simulink library "BicopLibrary"  (R2022b)
settings: Solver=VariableStepAuto  StartTime=0.0  StopTime=10.0  RelTol=1e-3
undefined symbols (not defined in the file or in its folder): Ts
libraries: arduinolib x7, $bdroot x3
settings Model: Creator=42190  LastModifiedBy=marti
settings DebuggingCC: UnconnectedInputMsg=warning  UnconnectedOutputMsg=warning  UnconnectedLineMsg=warning
settings ModelReferenceCC: EnableRefExpFcnMdlSchedulingChecks=on
settings RTWCC: DLArmComputeVersion=19.05

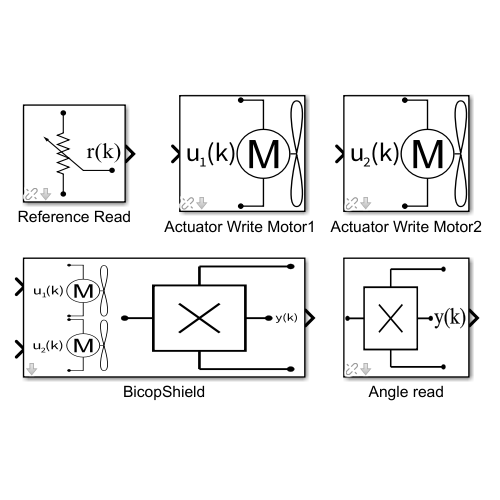
[thumbnail: Simulink's stored preview of the top-level diagram]
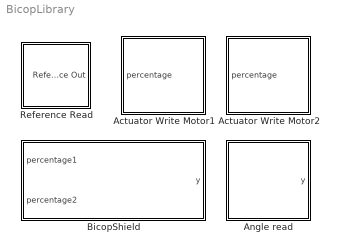
== system BicopLibrary ==
  "Actuator Write Motor1 " : Subsystem  AncestorBlock=BiCopLibrary/AeroShield/Actuator write
      settings: LibrarySourceBlock=BiCopLibrary/AeroShield/Actuator write
      mask DialogControl DescGroupVar Prompt: BicopShield actuator1
      mask DialogControl DescTextVar Prompt: Sets speed level to the first motor of the BicopShield. Expects input in form of percentual value from 0% to 100%.
      mask Display: image('$imagefile'); % Use "Edit Image" on toolstrip to change.
  Actuator Write Motor2 : Subsystem  AncestorBlock=BiCopLibrary/Actuator Write
      settings: LibrarySourceBlock=BiCopLibrary/Actuator Write
      mask DialogControl DescGroupVar Prompt: BicopShield actuator2
      mask DialogControl DescTextVar Prompt: Sets speed level to the second motor of the BicopShield. Expects input in form of percentual value from 0% to 100%.
      mask Display: image('$imagefile'); % Use "Edit Image" on toolstrip to change.
  Angle read : Subsystem  AncestorBlock=AeroLibrary/Angle read
      settings: LibrarySourceBlock=AeroLibrary/Angle read
      mask DialogControl DescGroupVar Prompt: BicopShield angle reading
      mask DialogControl DescTextVar Prompt: Sends commands to AS5600 sensor to read the pendulum angle. Output is in radians
      mask Display: image('$imagefile'); % Use "Edit Image" on toolstrip to change.
  BicopShield : Subsystem
      mask DialogControl DescGroupVar Prompt: BicopShield
      mask DialogControl DescTextVar Prompt: This block represents the BicopShield device. It accepts an input signal for powering the motors in the range of 0-100% and outputs a sensor angle reading in radians. Inside this system, you will find three subsystems. One of them reads the angle from sensor and the second one controls the BicopShield actuators respectively.
      mask Display: image('$imagefile'); % Use "Edit Image" on toolstrip to change.
  Reference Read : Subsystem  AncestorBlock=MotoLibrary/Reference Read
      settings: LibrarySourceBlock=MotoLibrary/Reference Read
      mask DialogControl DescGroupVar Prompt: BicopShield Potentiometer
      mask DialogControl DescTextVar Prompt: This blocks reads potentiometer wiper value on the BicopShield device. Return a percentage value.
      mask Display: image('$imagefile'); % Use "Edit Image" on toolstrip to change.

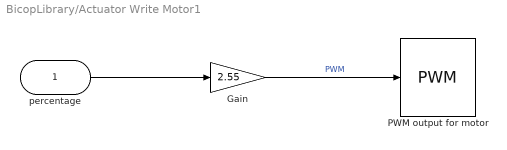
== system BicopLibrary/Actuator Write Motor1  ==
  percentage : Inport
  Gain : Gain  Gain=2.55
  "PWM output for motor " : arduinolib/PWM  pinNumber=5  frequencyType=Default  desiredFrequency=490.2  achievableFrequency=490.2
  wires:
  percentage/1 -> Gain/1
  Gain/1 -> "PWM output for motor "/1  "PWM"

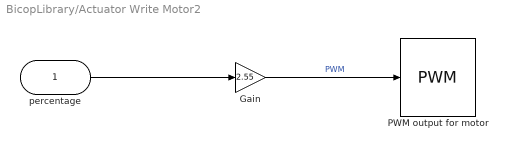
== system BicopLibrary/Actuator Write Motor2 ==
  percentage : Inport
  Gain : Gain  Gain=2.55
  "PWM output for motor " : arduinolib/PWM  pinNumber=6  frequencyType=Default  desiredFrequency=490.2  achievableFrequency=490.2
  wires:
  percentage/1 -> Gain/1
  Gain/1 -> "PWM output for motor "/1  "PWM"

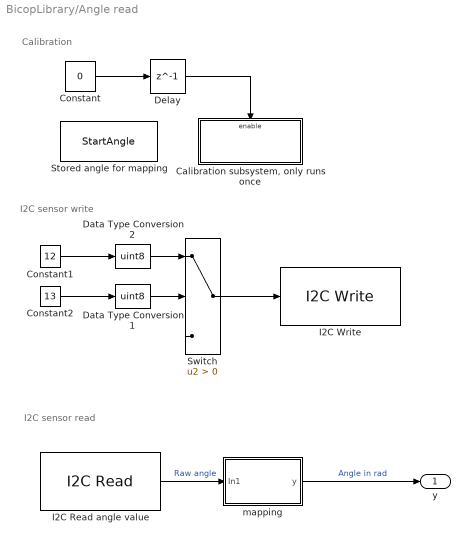
== system BicopLibrary/Angle read ==
  note: I2C sensor read
  note: I2C sensor write
  note: Calibration
  "Calibration subsystem, only runs once" : Subsystem  TreatAsAtomicUnit=on
  Constant : Constant  Value=0
  Constant1 : Constant  Value=12
  Constant2 : Constant  Value=13
  Data Type Conversion1 : DataTypeConversion  OutDataTypeStr=uint8  SaturateOnIntegerOverflow=off  RndMeth=Floor
  Data Type Conversion2 : DataTypeConversion  OutDataTypeStr=uint8  SaturateOnIntegerOverflow=off  RndMeth=Floor
  Delay : Delay  DelayLength=1  InitialCondition=1
  I2C Read angle value : arduinolib/I2C Read  I2CModule=0  Mode=Master  SlaveAddress=uint8(hex2dec('36'))  SlaveByteOrder=BigEndian  Direction=Receiver  RegisterAddressMode=off  RegisterAddress=uint8(hex2dec('36'))  SlaveDataType=uint16  DataLength=1  NoAck=off  RepeatedStart=off  OutputStatus=off  blockPlatform=ARDUINO  SampleTime=-1
  I2C Write : arduinolib/I2C Write  I2CModule=0  Mode=Master  SlaveAddress=uint8(hex2dec('36'))  SlaveByteOrder=BigEndian  Direction=Transmitter  RegisterAddressMode=off  RegisterAddress=uint8(hex2dec('0c'))  SlaveDataType=uint8  DataLength=1  NoAck=off  RepeatedStart=off  OutputStatus=off  blockPlatform=ARDUINO
  Stored angle for mapping : DataStoreMemory  DataStoreName=StartAngle  ReadBeforeWriteMsg=warning  WriteAfterWriteMsg=warning  WriteAfterReadMsg=warning  ShowAdditionalParam=off
  Switch : Switch  Criteria=u2 > Threshold  SaturateOnIntegerOverflow=off  InputSameDT=off
  mapping : Subsystem
  y : Outport
  wires:
  mapping/1(y) -> y/1  "Angle in rad"
  Constant/1 -> Delay/1
  Delay/1 -> "Calibration subsystem, only runs once"/Enable
  I2C Read angle value/1 -> mapping/1(In1)  "Raw angle"
  ? -> Switch/3
  Constant1/1 -> Data Type Conversion2/1
  Constant2/1 -> Data Type Conversion1/1
  Switch/1 -> I2C Write/1
  Data Type Conversion2/1 -> Switch/1
  Data Type Conversion1/1 -> Switch/2

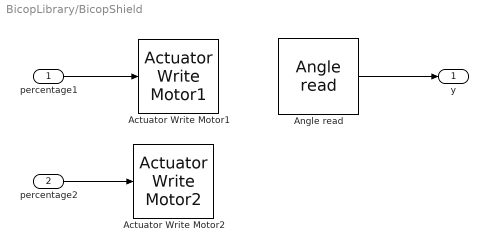
== system BicopLibrary/BicopShield ==
  percentage1 : Inport
  percentage2 : Inport  Port=2
  "Actuator Write Motor1 " : $bdroot/Actuator Write Motor1 
      settings: LibrarySourceBlock=BiCopLibrary/AeroShield/Actuator write
  Actuator Write Motor2 : $bdroot/Actuator Write Motor2
      settings: LibrarySourceBlock=BiCopLibrary/Actuator Write
  Angle read : $bdroot/Angle read
      settings: LibrarySourceBlock=AeroLibrary/Angle read
  y : Outport
  wires:
  percentage1/1 -> "Actuator Write Motor1 "/1
  Angle read/1 -> y/1
  percentage2/1 -> Actuator Write Motor2/1

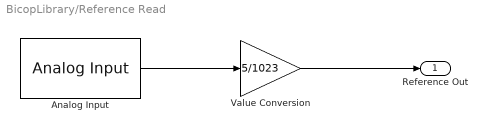
== system BicopLibrary/Reference Read ==
  Analog Input : arduinolib/Analog Input  pinNumber=3  ReadResultsOnly=off  ConversionTriggerSource=Software  ExternalTriggerType=uint32(0)  OutputDataType=uint16  EnableConversionCompleteNotify=off  EnableOuputStatus=off  SampleTime=Ts  blockPlatform=arduino
  Value Conversion : Gain  Gain=5/1023
  Reference Out : Outport
  wires:
  Analog Input/1 -> Value Conversion/1
  Value Conversion/1 -> Reference Out/1

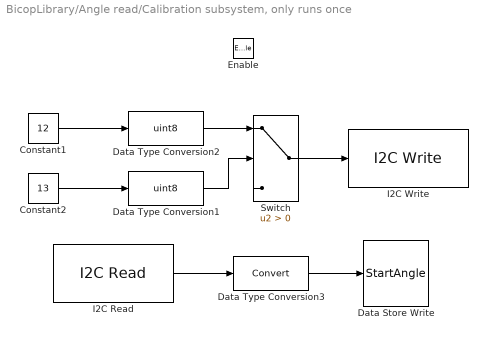
== system BicopLibrary/Angle read/Calibration subsystem, only runs once ==
  Enable : EnablePort
  Constant1 : Constant  Value=12
  Constant2 : Constant  Value=13
  Data Store Write : DataStoreWrite  DataStoreName=StartAngle  IndexOptions=Index vector (dialog)  Indices=1  OutputSizes=1
  Data Type Conversion1 : DataTypeConversion  OutDataTypeStr=uint8  SaturateOnIntegerOverflow=off  RndMeth=Floor
  Data Type Conversion2 : DataTypeConversion  OutDataTypeStr=uint8  SaturateOnIntegerOverflow=off  RndMeth=Floor
  Data Type Conversion3 : DataTypeConversion  SaturateOnIntegerOverflow=off  RndMeth=Floor
  I2C Read : arduinolib/I2C Read  I2CModule=0  Mode=Master  SlaveAddress=uint8(hex2dec('36'))  SlaveByteOrder=BigEndian  Direction=Receiver  RegisterAddressMode=off  RegisterAddress=uint8(hex2dec('36'))  SlaveDataType=uint16  DataLength=1  NoAck=off  RepeatedStart=off  OutputStatus=off  blockPlatform=ARDUINO  SampleTime=-1
  I2C Write : arduinolib/I2C Write  I2CModule=0  Mode=Master  SlaveAddress=uint8(hex2dec('36'))  SlaveByteOrder=BigEndian  Direction=Transmitter  RegisterAddressMode=off  RegisterAddress=uint8(hex2dec('0c'))  SlaveDataType=uint8  DataLength=1  NoAck=off  RepeatedStart=off  OutputStatus=off  blockPlatform=ARDUINO
  Switch : Switch  Criteria=u2 > Threshold  SaturateOnIntegerOverflow=off  InputSameDT=off
  wires:
  Constant2/1 -> Data Type Conversion1/1
  I2C Read/1 -> Data Type Conversion3/1
  Data Type Conversion2/1 -> Switch/1
  Data Type Conversion1/1 -> Switch/2
  Constant1/1 -> Data Type Conversion2/1
  Switch/1 -> I2C Write/1
  Data Type Conversion3/1 -> Data Store Write/1

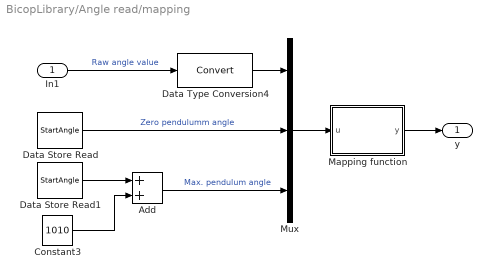
== system BicopLibrary/Angle read/mapping ==
  In1 : Inport
  Add : Sum
  Constant3 : Constant  Value=1010
  Data Store Read : DataStoreRead  DataStoreName=StartAngle  IndexOptions=Index vector (dialog)  Indices=1  OutputSizes=1
  Data Store Read1 : DataStoreRead  DataStoreName=StartAngle  IndexOptions=Index vector (dialog)  Indices=1  OutputSizes=1
  Data Type Conversion4 : DataTypeConversion  SaturateOnIntegerOverflow=off  RndMeth=Floor
  Mapping function : MATLAB Function  TreatAsAtomicUnit=on
  Mux : Mux  Inputs=3
  y : Outport
  wires:
  Constant3/1 -> Add/2
  Data Store Read/1 -> Mux/2  "Zero pendulumm angle"
  In1/1 -> Data Type Conversion4/1  "Raw angle value"
  Add/1 -> Mux/3  "Max. pendulum angle"
  Mapping function/1(y) -> y/1
  Data Store Read1/1 -> Add/1
  Mux/1 -> Mapping function/1(u)
  Data Type Conversion4/1 -> Mux/1

== matlab function BicopLibrary/Angle read/mapping/Mapping function ==
  data: u input; y output
function y = fcn(u)
angMin=0;
angMax=1.55;
y = ((u(1) - u(2)) * (angMax - angMin)) / (u(3) - u(2)) + angMin ;
